simulink library "pct23_lib"  (R2018b)
settings: Solver=VariableStepAuto  StartTime=0.0  StopTime=10.0  RelTol=1e-3
settings Model: Creator=MK  LastModifiedBy=MK

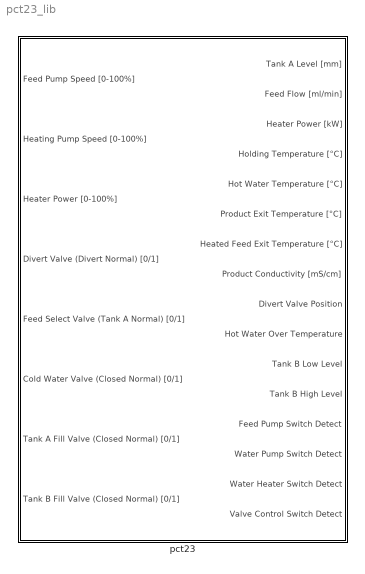
== system pct23_lib ==
  pct23 : Subsystem

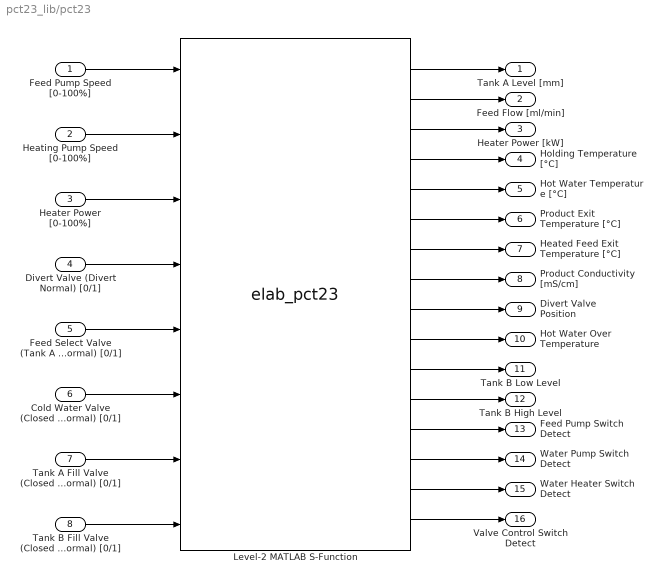
== system pct23_lib/pct23 ==
  Feed Pump Speed [0-100%] : Inport
  Heating Pump Speed [0-100%] : Inport  Port=2
  Heater Power [0-100%] : Inport  Port=3
  Divert Valve (Divert Normal) [0/1] : Inport  Port=4
  Feed Select Valve (Tank A Normal) [0/1] : Inport  Port=5
  Cold Water Valve (Closed Normal) [0/1] : Inport  Port=6
  Tank A Fill Valve (Closed Normal) [0/1] : Inport  Port=7
  Tank B Fill Valve (Closed Normal) [0/1] : Inport  Port=8
  Level-2 MATLAB S-Function : M-S-Function  FunctionName=elab_pct23  Parameters=Ts, address, logging
  Tank A Level [mm] : Outport
  Feed Flow [ml/min] : Outport  Port=2
  Heater Power [kW] : Outport  Port=3
  Holding Temperature [°C] : Outport  Port=4
  Hot Water Temperature [°C] : Outport  Port=5
  Product Exit Temperature [°C] : Outport  Port=6
  Heated Feed Exit Temperature [°C] : Outport  Port=7
  Product Conductivity [mS/cm] : Outport  Port=8
  Divert Valve Position : Outport  Port=9
  Hot Water Over Temperature : Outport  Port=10
  Tank B Low Level : Outport  Port=11
  Tank B High Level : Outport  Port=12
  Feed Pump Switch Detect : Outport  Port=13
  Water Pump Switch Detect : Outport  Port=14
  Water Heater Switch Detect : Outport  Port=15
  Valve Control Switch Detect : Outport  Port=16
  wires:
  Divert Valve (Divert Normal) [0/1]/1 -> Level-2 MATLAB S-Function/4
  Level-2 MATLAB S-Function/9 -> Divert Valve Position/1
  Level-2 MATLAB S-Function/13 -> Feed Pump Switch Detect/1
  Feed Pump Speed [0-100%]/1 -> Level-2 MATLAB S-Function/1
  Level-2 MATLAB S-Function/6 -> Product Exit Temperature [°C]/1
  Level-2 MATLAB S-Function/7 -> Heated Feed Exit Temperature [°C]/1
  Level-2 MATLAB S-Function/14 -> Water Pump Switch Detect/1
  Level-2 MATLAB S-Function/11 -> Tank B Low Level/1
  Level-2 MATLAB S-Function/4 -> Holding Temperature [°C]/1
  Level-2 MATLAB S-Function/8 -> Product Conductivity [mS/cm]/1
  Cold Water Valve (Closed Normal) [0/1]/1 -> Level-2 MATLAB S-Function/6
  Level-2 MATLAB S-Function/12 -> Tank B High Level/1
  Level-2 MATLAB S-Function/10 -> Hot Water Over Temperature/1
  Level-2 MATLAB S-Function/16 -> Valve Control Switch Detect/1
  Level-2 MATLAB S-Function/15 -> Water Heater Switch Detect/1
  Heating Pump Speed [0-100%]/1 -> Level-2 MATLAB S-Function/2
  Heater Power [0-100%]/1 -> Level-2 MATLAB S-Function/3
  Feed Select Valve (Tank A Normal) [0/1]/1 -> Level-2 MATLAB S-Function/5
  Tank B Fill Valve (Closed Normal) [0/1]/1 -> Level-2 MATLAB S-Function/8
  Tank A Fill Valve (Closed Normal) [0/1]/1 -> Level-2 MATLAB S-Function/7
  Level-2 MATLAB S-Function/1 -> Tank A Level [mm]/1
  Level-2 MATLAB S-Function/3 -> Heater Power [kW]/1
  Level-2 MATLAB S-Function/2 -> Feed Flow [ml/min]/1
  Level-2 MATLAB S-Function/5 -> Hot Water Temperature [°C]/1
